simulink model "New_Prandtl"  (Simulink 7.9)
settings: Solver=FixedStepDiscrete  StartTime=0.0  StopTime=10  FixedStep=1  RelTol=1e-3
undefined symbols (not defined in the file): Carnot_Prandtl_Callbacks
settings Model: Creator=awohlfei  LastModifiedBy=awohlfei

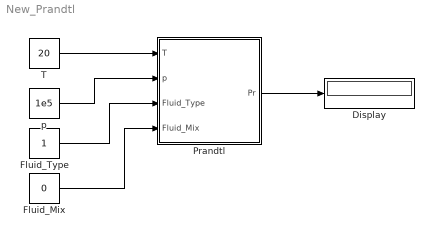
== system New_Prandtl ==
  Display : Display
  Fluid_Mix : Constant  Value=0
  Fluid_Type : Constant
  Prandtl : Subsystem  LoadFcn=Carnot_Prandtl_Callbacks('LoadFcn');  InitFcn=load('THB.mat');  VariantObject=CarlibClassic  mask(Prandtl){INPUTARGUMENTS=state variables (classic), DEBUGLEVEL=WARNING, MAXTOTALMESSAGES=inf, MAXCONSECUTIVEMESSAGES=inf, WRITETOFILE=0, FILENAME='errors.txt'}
      mask prompts: INPUTARGUMENTS "Input arguments"; DEBUGLEVEL "Debug level"; MAXTOTALMESSAGES "maximum number of total warning"; MAXCONSECUTIVEMESSAGES "maximum number of consecutive warnings"; WRITETOFILE "write messages to file"; FILENAME "filename for error messages"
      mask help:
      | Calculates the Prandtl number for given materials properties.
      | Definition of the fluid types
      |  1        water
      |  2        air                    fluid_mix is (kg water) / (kg air)
      |  3        cotton oil
      |  4        silicone oil
      |  5        water-glycol    fluid_mix gives the volume-percent of glycol
      |  6        tyfocor LS      only available in liquid phase
      mask init:
      | %Inports
      | Carnot_Prandtl_Callbacks('CreateInports');
      | 
      | %global debug level
      | [DEBUGLEVEL, MAXTOTALMESSAGES, MAXCONSECUTIVEMESSAGES, WRITETOFILE, FILENAME] = Carnot_Prandtl_Callbacks('CheckDebugLevels', DEBUGLEVEL, MAXTOTALMESSAGES, MAXCONSECUTIVEMESSAGES, WRITETOFILE, FILENAME);
      mask Help: eval('man(''prandtl'')')
      mask StyleString: popup(state variables (classic)|THB|THV),popup(DEBUG|INFO|WARNING|ERROR|FATAL|NONE),edit,edit,edit,edit
      mask CallbackString: Carnot_Prandtl_Callbacks('MaskVisibilities');|||||
      mask TabNameString: Parameters,Debugging,Debugging,Debugging,Debugging,Debugging
  T : Constant  Value=20
  p : Constant  Value=1e5
  wires:
  T/1 -> Prandtl/1(T)
  p/1 -> Prandtl/2(p)
  Fluid_Type/1 -> Prandtl/3(Fluid_Type)
  Fluid_Mix/1 -> Prandtl/4(Fluid_Mix)
  Prandtl/1(Pr) -> Display/1

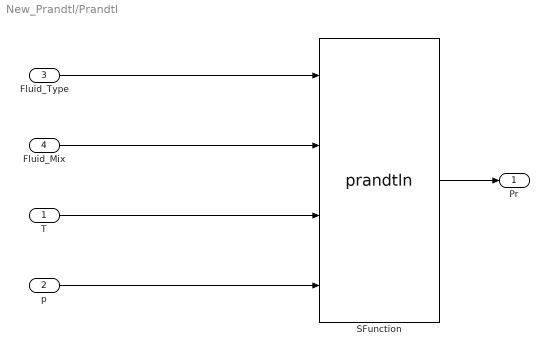
== system New_Prandtl/Prandtl ==
  T : Inport
  p : Inport  Port=2
  Fluid_Type : Inport  Port=3
  Fluid_Mix : Inport  Port=4
  SFunction : S-Function  FunctionName=prandtln  Parameters=DEBUGLEVEL,MAXTOTALMESSAGES,MAXCONSECUTIVEMESSAGES,WRITETOFILE,FILENAME  EnableBusSupport=off
  Pr : Outport
  wires:
  SFunction/1 -> Pr/1
  T/1 -> SFunction/3
  p/1 -> SFunction/4
  Fluid_Type/1 -> SFunction/1
  Fluid_Mix/1 -> SFunction/2
